simulink model "benuoc"  (R2018a)
settings: Solver=ode5  StartTime=0.0  StopTime=1000  FixedStep=1  RelTol=1e-3
undefined symbols (not defined in the file): sigbuilder_block
libraries: fuzblock x1
settings Model: Creator=DELL  LastModifiedBy=DELL

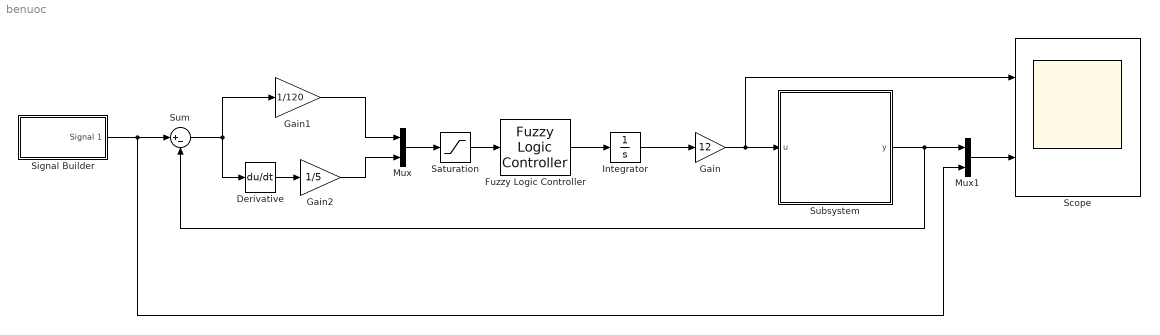
== system benuoc ==
  Derivative : Derivative
  Fuzzy Logic Controller : fuzblock/Fuzzy Logic  Controller  FIS='fuzzy1.fis'  OutputSampleNumber=101  DataType=double  FuzzifiedInputs=off  RuleFiringStrengths=off  RuleOutputs=off  AggregatedOutputs=off  SimulateUsing=Interpreted execution  OutOfRangeInputValueMessage=warning  NoRuleFiredMessage=warning  EmptyOutputFuzzySetMessage=warning
  Gain : Gain  Gain=12
  Gain1 : Gain  Gain=1/120
  Gain2 : Gain  Gain=1/5
  Integrator : Integrator  LimitOutput=on  UpperSaturationLimit=1  LowerSaturationLimit=0
  Mux : Mux  Inputs=2
  Mux1 : Mux  Inputs=2
  Saturation : Saturate  UpperLimit=1  LowerLimit=-1
  Scope : Scope  NumInputPorts=2
  Signal Builder : Subsystem  Tag=STV Subsys  LoadFcn=sigbuilder_block('load');  StartFcn=sigbuilder_block('start');  StopFcn=sigbuilder_block('stop');  ClipboardFcn=sigbuilder_block('clipboard');  mask(Sigbuilder block){tuvar=[0:10]}
      mask help: Simulink:masks:SigbuilderBlock_MD
      mask init:
      | if ~strcmp(get_param(bdroot(gcbh),'SimulationStatus'),'stopped') tuvar = sigbuilder_block('maskInit'); end
      settings: CopyFcn=sigbuilder_block('copy');  DeleteFcn=sigbuilder_block('delete');  ModelCloseFcn=sigbuilder_block('modelClose');  PreSaveFcn=sigbuilder_block('preSave');  PauseFcn=sigbuilder_block('pause');  ContinueFcn=sigbuilder_block('continue');  NameChangeFcn=sigbuilder_block('namechange');  OpenFcn=sigbuilder_block('open',[395.4 115.8 550.8 400.2 ]);  CloseFcn=sigbuilder_block('close');
      mask Display: plot(0, 0, 100, 100,[2, 2, 32, 32, 2], [68, 8, 8, 68, 68],[32, 2], [38, 38], [32, 19, 2],[53, 60, 44], [32, 17, 17, 2],[16, 16, 31, 31]);txt = getActiveGroup(gcbh);text(2, 100, txt,'verticalAlignment', 'top');
  Subsystem : Subsystem  mask{A=200, b=1.5, C=0.8, k=60, g=981}
  Sum : Sum  Inputs=|+-
  wires:
  Fuzzy Logic Controller/1 -> Integrator/1
  Mux/1 -> Saturation/1
  Gain1/1 -> Mux/1
  Gain2/1 -> Mux/2
  Sum/1 -> Gain1/1, Derivative/1
  Derivative/1 -> Gain2/1
  Gain/1 -> Scope/1, Subsystem/1(u)
  Signal Builder/1(Signal 1) -> Mux1/2, Sum/1
  Integrator/1 -> Gain/1
  Subsystem/1(y) -> Sum/2, Mux1/1
  Mux1/1 -> Scope/2
  Saturation/1 -> Fuzzy Logic Controller/1

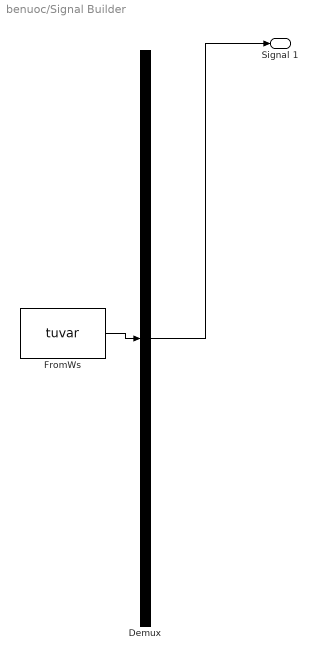
== system benuoc/Signal Builder ==
  Demux : Demux  Tag=STV Demux  Outputs=1
  FromWs : FromWorkspace  Tag=STV FromWs  VariableName=tuvar  SampleTime=0
      SigBuilderData=|
      | common.afterFinalStr = 'Extrapolate'
      | common.sampleTime = 0
      | dataSet.timeRange = [0 1000]
      | dataSet.name = 'Group 1'
      | sbobj.Groups.Name = 'Group 1'
      | sbobj.Groups.Signals.Name = 'Signal 1'
      | sbobj.Groups.Signals.XData = [0 202 202 400 400 598 598 804 804 1000]
      | sbobj.Groups.Signals.YData = [73.4 73.4 120.2 120.2 85.6 85.6 49.5 49.5 95.8 95.8]
      | sbobj.Groups.TimeRange = [0 1000]
  Signal 1 : Outport  Tag=STV Outport
  wires:
  Demux/1 -> Signal 1/1
  FromWs/1 -> Demux/1

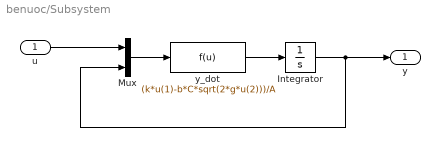
== system benuoc/Subsystem ==
  u : Inport
  Integrator : Integrator
  Mux : Mux  Inputs=2
  y_dot : Fcn  Expr=(k*u(1)-b*C*sqrt(2*g*u(2)))/A
  y : Outport
  wires:
  y_dot/1 -> Integrator/1
  Integrator/1 -> y/1, Mux/2
  u/1 -> Mux/1
  Mux/1 -> y_dot/1
